simulink model "untitled"  (R2018b)
settings: Solver=ode23  StartTime=0.0  StopTime=48  RelTol=1e-3
libraries: simulink x5
settings Model: Creator=Yogesh  LastModifiedBy=Yogesh

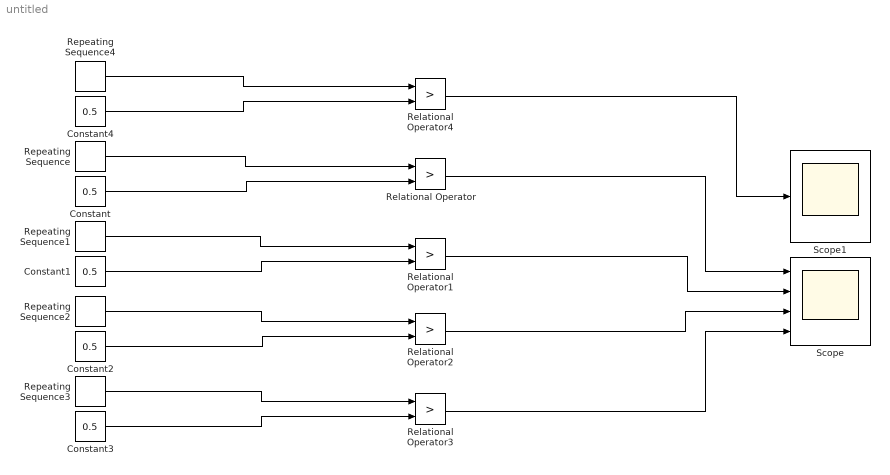
== system untitled ==
  Constant{,1..4} (5 alike) : Constant  Value=0.5
  Relational Operator{,1..4} (5 alike) : RelationalOperator  Operator=>  OutDataTypeStr=boolean  RndMeth=Simplest
  Repeating Sequence : simulink/Sources/Repeating Sequence  rep_seq_t=t  rep_seq_y=sig1
  Repeating Sequence1 : simulink/Sources/Repeating Sequence  rep_seq_t=t  rep_seq_y=sig2
  Repeating Sequence2 : simulink/Sources/Repeating Sequence  rep_seq_t=t  rep_seq_y=sig3
  Repeating Sequence3 : simulink/Sources/Repeating Sequence  rep_seq_t=t  rep_seq_y=sig4
  Repeating Sequence4 : simulink/Sources/Repeating Sequence  rep_seq_t=t  rep_seq_y=clk
  Scope : Scope  NumInputPorts=4
  Scope1 : Scope
  wires:
  Repeating Sequence/1 -> Relational Operator/1
  Relational Operator/1 -> Scope/1
  Constant/1 -> Relational Operator/2
  Repeating Sequence1/1 -> Relational Operator1/1
  Constant1/1 -> Relational Operator1/2
  Relational Operator1/1 -> Scope/2
  Repeating Sequence2/1 -> Relational Operator2/1
  Constant2/1 -> Relational Operator2/2
  Relational Operator2/1 -> Scope/3
  Repeating Sequence3/1 -> Relational Operator3/1
  Constant3/1 -> Relational Operator3/2
  Relational Operator3/1 -> Scope/4
  Repeating Sequence4/1 -> Relational Operator4/1
  Constant4/1 -> Relational Operator4/2
  Relational Operator4/1 -> Scope1/1
